simulink model "Medium_Intro_Lab"  (R2021a)
settings: Solver=VariableStepAuto  StartTime=0.0  StopTime=10.0  MaxStep=1e-3  RelTol=1e-3
libraries: simulink x1
settings Model: Creator=reemb  LastModifiedBy=reemb

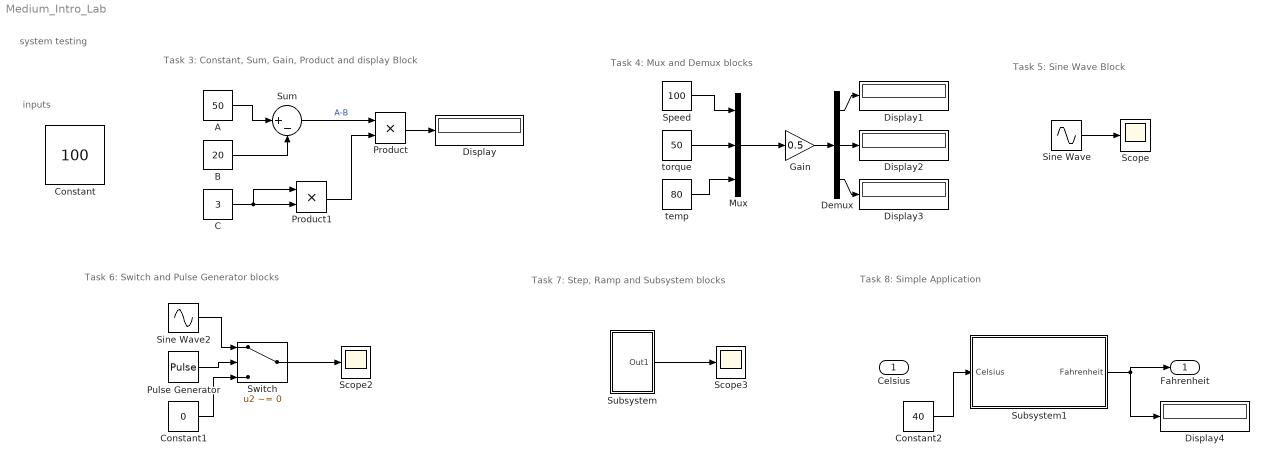
== system Medium_Intro_Lab ==
  note: Task 5: Sine Wave Block
  note: Task 4: Mux and Demux blocks
  note: Task 3: Constant, Sum, Gain, Product and display Block
  note: system testing
  note: inputs
  note: Task 8: Simple Application
  note: Task 6: Switch and Pulse Generator blocks
  note: Task 7: Step, Ramp and Subsystem blocks
  Celsius : Inport
  A : Constant  Value=50
  B : Constant  Value=20
  C : Constant  Value=3
  Constant : Constant  Value=100
  Constant1 : Constant  Value=0
  Constant2 : Constant  Value=40
  Demux : Demux  Outputs=3
  Display{,1..4} (5 alike) : Display
  Gain : Gain  Gain=0.5
  Mux : Mux  Inputs=3
  Product : Product
  Product1 : Product
  Pulse Generator : DiscretePulseGenerator  PulseType=Time based  PulseWidth=50
  Scope : Scope
  Scope2 : Scope
  Scope3 : Scope
  Sine Wave : Sin  Amplitude=10  Frequency=5  Phase=pi/2  SampleTime=0
  Sine Wave2 : Sin  Amplitude=5  Frequency=10  SampleTime=0
  Speed : Constant  Value=100
  Subsystem : Subsystem
  Subsystem1 : Subsystem
  Sum : Sum  Inputs=|+-
  Switch : Switch  Criteria=u2 ~= 0
  temp : Constant  Value=80
  torque : Constant  Value=50
  Fahrenheit : Outport
  wires:
  A/1 -> Sum/1
  B/1 -> Sum/2
  Sum/1 -> Product/1  "A-B"
  C/1 -> Product1/1, Product1/2
  Product1/1 -> Product/2
  Product/1 -> Display/1
  Speed/1 -> Mux/1
  torque/1 -> Mux/2
  Mux/1 -> Gain/1
  temp/1 -> Mux/3
  Gain/1 -> Demux/1
  Demux/1 -> Display1/1
  Demux/2 -> Display2/1
  Demux/3 -> Display3/1
  Sine Wave/1 -> Scope/1
  Sine Wave2/1 -> Switch/1
  Constant1/1 -> Switch/3
  Pulse Generator/1 -> Switch/2
  Switch/1 -> Scope2/1
  Subsystem/1(Out1) -> Scope3/1
  Subsystem1/1(Fahrenheit) -> Fahrenheit/1, Display4/1
  Constant2/1 -> Subsystem1/1(Celsius)

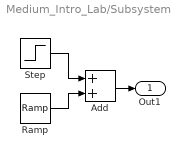
== system Medium_Intro_Lab/Subsystem ==
  Add : Sum
  Ramp : simulink/Sources/Ramp  slope=3  start=2  InitialOutput=0
  Step : Step  Time=2  After=5  SampleTime=0
  Out1 : Outport
  wires:
  Step/1 -> Add/1
  Ramp/1 -> Add/2
  Add/1 -> Out1/1

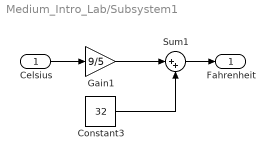
== system Medium_Intro_Lab/Subsystem1 ==
  Celsius : Inport
  Constant3 : Constant  Value=32
  Gain1 : Gain  Gain=9/5
  Sum1 : Sum  Inputs=|++
  Fahrenheit : Outport
  wires:
  Celsius/1 -> Gain1/1
  Constant3/1 -> Sum1/2
  Gain1/1 -> Sum1/1
  Sum1/1 -> Fahrenheit/1
